simulink model "lidar_webcam_SGcomV6"  (Simulink 7.3)
settings: Solver=FixedStepDiscrete  StartTime=0.0  StopTime=inf  MaxStep=0.2  RelTol=1e-3
settings Model: Creator=gclayton  LastModifiedBy=wildcat
settings DebuggingCC: InheritedTsInSrcMsg=none
settings RTWCC: SystemTargetFile=rlnx.tlc  GenCodeOnly=on  TemplateMakefile=rlnx_ubuntu.tmf  Description=Linux Real-Time Target  ProcessScript=rlnx_make_rtw_hook
settings RTWCC: CustomInclude=|
  | /usr/local/include/opencv/
  | /usr/local/include/
settings CodeAppCC: GenerateComments=off  SimulinkBlockComments=off
settings STFCustomTargetCC: ModelReferenceCompliant=off  MatFileLogging=on  SystemTargetFile=rlnx.tlc
settings GRTTargetCC: ModelReferenceCompliant=off  ParMdlRefBuildCompliant=off  CompOptLevelCompliant=off
settings CustomProperty: DataType=string  Value=-lm -ldl /usr/local/lib/libopencv_highgui.so.2.4 /usr/local/lib/libopencv_core.so.2.4 /usr/local/lib/libopencv_imgproc.so.2.4 -lc_urg -lc_urg_connection -lc_urg_system -lphidget21
settings EnumStrPairs: String=PC

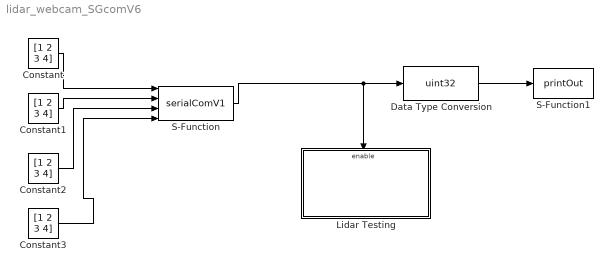
== system lidar_webcam_SGcomV6 ==
  Constant : Constant  Value=[1 2 3 4]  VectorParams1D=off  OutDataTypeMode=double  OutDataType=fixdt(1, 16)  OutScaling=2^0  OutDataTypeStr=double
  Constant1 : Constant  Value=[1 2 3 4]  VectorParams1D=off  OutDataTypeMode=int32  OutDataType=fixdt(1, 16)  OutScaling=2^0  OutDataTypeStr=int32
  Constant2 : Constant  Value=[1 2 3 4]  VectorParams1D=off  OutDataTypeMode=int32  OutDataType=fixdt(1, 16)  OutScaling=2^0  OutDataTypeStr=int32
  Constant3 : Constant  Value=[1 2 3 4]  VectorParams1D=off  OutDataTypeMode=int32  OutDataType=fixdt(1, 16)  OutScaling=2^0  OutDataTypeStr=int32
  Data Type Conversion : DataTypeConversion  OutDataTypeMode=uint32  OutDataType=fixdt(1, 16)  OutScaling=2^0  OutDataTypeStr=uint32
  Lidar Testing : Subsystem  TreatAsAtomicUnit=on
  S-Function : S-Function  FunctionName=serialComV1  EnableBusSupport=off
  S-Function1 : S-Function  FunctionName=printOut  EnableBusSupport=off
  wires:
  S-Function/1 -> Lidar Testing/Enable, Data Type Conversion/1
  Constant/1 -> S-Function/1
  Constant1/1 -> S-Function/2
  Constant2/1 -> S-Function/3
  Constant3/1 -> S-Function/4
  Data Type Conversion/1 -> S-Function1/1

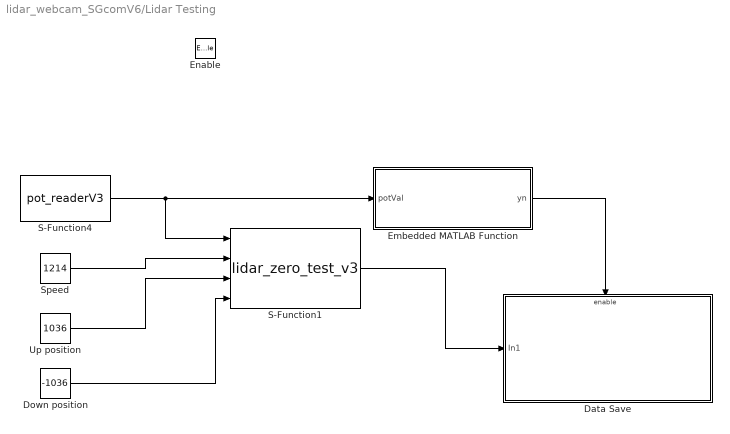
== system lidar_webcam_SGcomV6/Lidar Testing ==
  Enable : EnablePort
  Data Save : Subsystem  TreatAsAtomicUnit=on
  Down position : Constant  Value=-1036  OutDataType=fixdt(1, 16)  OutScaling=2^0
  Embedded MATLAB Function : Stateflow chart
  S-Function1 : S-Function  FunctionName=lidar_zero_test_v3  EnableBusSupport=off
  S-Function4 : S-Function  FunctionName=pot_readerV3  EnableBusSupport=off
  Speed : Constant  Value=1214  OutDataType=fixdt(1, 16)  OutScaling=2^0
  Up position : Constant  Value=1036  OutDataType=fixdt(1, 16)  OutScaling=2^0
  wires:
  Speed/1 -> S-Function1/2
  Up position/1 -> S-Function1/3
  Down position/1 -> S-Function1/4
  S-Function4/1 -> S-Function1/1, Embedded MATLAB Function/1(potVal)
  S-Function1/1 -> Data Save/1(In1)
  Embedded MATLAB Function/1(yn) -> Data Save/Enable

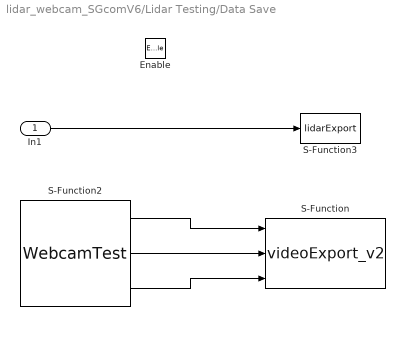
== system lidar_webcam_SGcomV6/Lidar Testing/Data Save ==
  In1 : Inport  OutDataType=fixdt(1, 16)  OutScaling=2^0
  Enable : EnablePort
  S-Function : S-Function  FunctionName=videoExport_v2  EnableBusSupport=off
  S-Function2 : S-Function  FunctionName=WebcamTest  EnableBusSupport=off
  S-Function3 : S-Function  FunctionName=lidarExport  EnableBusSupport=off
  wires:
  S-Function2/3 -> S-Function/3
  S-Function2/2 -> S-Function/2
  S-Function2/1 -> S-Function/1
  In1/1 -> S-Function3/1

== matlab function Lidar Testing/Embedded MATLAB Function ==
  data: potVal input double; yn output double
function yn = check_pot_val(potVal)
%#eml

% Pot value may initially be zero.
% Check for this and output a 1 or zero to 
% control whether the rest of model runs
if (potVal == 0)
    yn = 0;
else
    yn = 1;
end
